simulink model "stm32f4_clcd_demo_4lines"  (Simulink 7.3)
settings: Solver=FixedStepDiscrete  SolverMode=SingleTasking  StartTime=0.0  StopTime=10.0  RelTol=1e-3
PreLoadFcn:
  | waijung.modelPreload; % Required for working with Waijung Blockset. Do not remove.
undefined symbols (not defined in the file): HSEOSC, Link, LQFP176, ST, STM32F417IG
libraries: simulink x1, stm32f4_adc_lib x1, stm32f4_device_config_lib x1
CloseFcn:
  | waijung.modelClose; % Required for working with Waijung Blockset. Do not remove.
settings Model: Creator=Krisada  LastModifiedBy=Krisada
settings OptimizationCC: OptimizeModelRefInitCode=on  LifeSpan=1
settings DebuggingCC: ParameterPrecisionLossMsg=none
settings HardwareCC: ProdEndianess=LittleEndian  ProdHWDeviceType=ARM Compatible->Cortex - M4  TargetEndianess=LittleEndian  TargetHWDeviceType=ARM Compatible->Cortex - M4
settings RTWCC: SystemTargetFile=stm32f4.tlc  GenerateMakefile=off  TemplateMakefile=ert_default_tmf  Description=STM32F4 Target  ProcessScript=stm32f4_make_rtw_hook
settings CodeAppCC: IgnoreCustomStorageClasses=off
settings STFCustomTargetCC: ModelReferenceCompliant=off  CombineOutputUpdateFcns=on  ERTCustomFileBanners=on  SupportContinuousTime=off  SupportNonInlinedSFcns=off  SystemTargetFile=stm32f4.tlc
settings ERTTargetCC: MultiwordLength=2048  ModelReferenceCompliant=off  ParMdlRefBuildCompliant=off  CompOptLevelCompliant=off  ERTFirstTimeCompliant=off  ModelStepFunctionPrototypeControlCompliant=off  CPPClassGenCompliant=off  ExtModeMexFile=noextcomm  InlinedParameterPlacement=NonHierarchical  ERTSrcFileBannerTemplate=stm32f4_code_template.cgt  ERTHdrFileBannerTemplate=stm32f4_code_template.cgt  ERTDataSrcFileTemplate=stm32f4_code_template.cgt  ERTDataHdrFileTemplate=stm32f4_code_template.cgt  ERTCustomFileTemplate=stm32f4_file_process.tlc

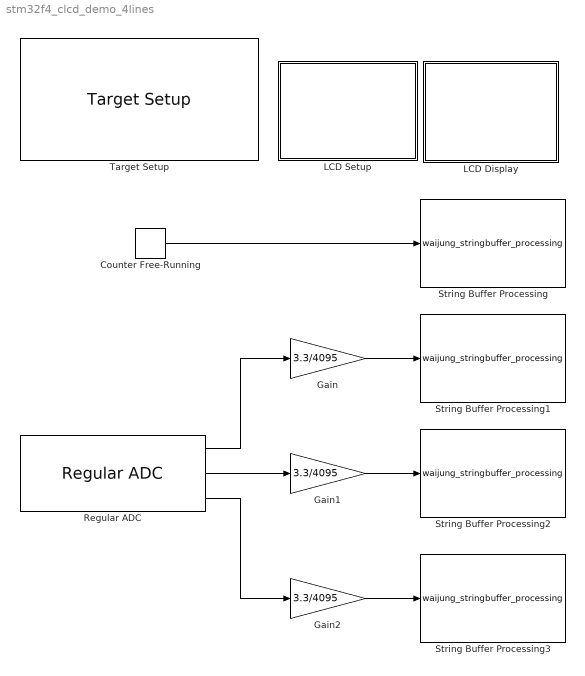
== system stm32f4_clcd_demo_4lines ==
  Counter Free-Running : simulink/Sources/Counter Free-Running  SystemSampleTime=-1  NumBits=16  tsamp=0.01
  Gain : Gain  Gain=3.3/4095  ParameterDataTypeMode=single  ParameterDataType=fixdt(1, 16)  ParameterScaling=2^0  ParamDataTypeStr=single  OutDataTypeMode=single  OutDataType=fixdt(1, 16)  OutScaling=2^0  OutDataTypeStr=single
  Gain1 : Gain  Gain=3.3/4095  ParameterDataTypeMode=single  ParameterDataType=fixdt(1, 16)  ParameterScaling=2^0  ParamDataTypeStr=single  OutDataTypeMode=single  OutDataType=fixdt(1, 16)  OutScaling=2^0  OutDataTypeStr=single
  Gain2 : Gain  Gain=3.3/4095  ParameterDataTypeMode=single  ParameterDataType=fixdt(1, 16)  ParameterScaling=2^0  ParamDataTypeStr=single  OutDataTypeMode=single  OutDataType=fixdt(1, 16)  OutScaling=2^0  OutDataTypeStr=single
  LCD Display : Subsystem
  LCD Setup : Subsystem
  Regular ADC : stm32f4_adc_lib/Regular ADC  adcmodule=1  outputdatatype=Single  prescaler=2  prescalerstr=ADC_Prescaler_Div2  chsamplingtime=Auto  chsamplingtimestr=ADC_SampleTime_480Cycles  read_an0=on  read_an1=on  read_an2=on  read_an3=off  read_an4=off  read_an5=off  read_an6=off  read_an7=off  read_an8=off  read_an9=off  read_an10=off  read_an11=off  read_an12=off  read_an13=off  read_an14=off  read_an15=off  read_an16=off  read_an17=off  read_an18=off  pinstr=GPIO_Pin_0 | GPIO_Pin_1 | GPIO_Pin_2  usedpinarray="[1  1  1  0  0  0  0  0  0  0  0  0  0  0  0  0  0  0  0]"  usedportidarray="[0  0  0]"  usedpinidarray="[0  1  2]"  usedpinidcount=3  sampletime=0.01  blockid=RegularADC  enablecustomportlabel=off  cinputportlabel=0  coutputportlabel=Out1, Out2
  String Buffer Processing : S-Function  FunctionName=waijung_stringbuffer_processing  Parameters=configuration,varname,sformat,porttypes,portcount,inputtypearray,outputtypearray,sampletime,sampletimestr,blockid  EnableBusSupport=off  mask(waijung_stringbuffer_processing){configuration=sprintf, storagename=Line1, sformat='Index: %u', enableoutput=off, varname=LCDSetupVolatileDataStorage_Line1, inputtypearray=[1 -1], outputtypearray=[0], porttypes=["uint32_t"], portcount=1, sampletime=-1, sampletimestr=0.01, blockid=StringBufferProcessing}
      mask prompts: configuration "Function"; storagename "String buffer"; sformat "Printf format"; enableoutput "Enable output status"; varname "Variable name"; inputtypearray "Input type array"; outputtypearray "Output type array"; porttypes "Port type list"; portcount "Port type count"; sampletime "Sample time (sec)"; sampletimestr "Compiled sample time (sec) in string"
      mask help:
      | This block implements string processing, sprintf/ sscanf command.
      | Supported format:
      | %u, %i, %o, %x: uint32
      | %d: int32
      | %e, %g, %f: single
      | %c: int8
      |
      | Status:
      |  0: Failed.
      |  Non-zero: Success.
      mask init:
      | waijung_stringbuffer_processing_callback('init');
      mask Help: web(fullfile(waijungdocroot,'String_Buffer_Processing.htm'))
      mask StyleString: popup(sprintf|sscanf),popup(Line1|Line2|Line3|Line4|<output>),edit,checkbox,edit,edit,edit,edit,edit,edit,edit,edit
      mask CallbackString: waijung_stringbuffer_processing_callback('configuration');||waijung_stringbuffer_processing_callback('sformat');|waijung_stringbuffer_processing_callback('enableoutput');||||||waijung_stringbuffer_processing_callback('sampletime');|waijung_stringbuffer_processing_callback('sampletimestr');|waijung_stringbuffer_processing_callback('blockid');
      mask Display: text(0.5, 0.5, '[ sprintf ]\nBuffer: Line1\nTs (sec): 0.01','ver','middle','hor','center');port_label('input', 1,'%u');
  String Buffer Processing1 : S-Function  FunctionName=waijung_stringbuffer_processing  Parameters=configuration,varname,sformat,porttypes,portcount,inputtypearray,outputtypearray,sampletime,sampletimestr,blockid  EnableBusSupport=off  mask(waijung_stringbuffer_processing){configuration=sprintf, storagename=Line2, sformat='AN0: %1.3f V', enableoutput=off, varname=LCDSetupVolatileDataStorage1_Line2, inputtypearray=[1 -1], outputtypearray=[0], porttypes=["float"], portcount=1, sampletime=-1, sampletimestr=0.01, blockid=StringBufferProcessing1}
      mask prompts: configuration "Function"; storagename "String buffer"; sformat "Printf format"; enableoutput "Enable output status"; varname "Variable name"; inputtypearray "Input type array"; outputtypearray "Output type array"; porttypes "Port type list"; portcount "Port type count"; sampletime "Sample time (sec)"; sampletimestr "Compiled sample time (sec) in string"
      mask help:
      | This block implements string processing, sprintf/ sscanf command.
      | Supported format:
      | %u, %i, %o, %x: uint32
      | %d: int32
      | %e, %g, %f: single
      | %c: int8
      |
      | Status:
      |  0: Failed.
      |  Non-zero: Success.
      mask init:
      | waijung_stringbuffer_processing_callback('init');
      mask Help: web(fullfile(waijungdocroot,'String_Buffer_Processing.htm'))
      mask StyleString: popup(sprintf|sscanf),popup(Line1|Line2|Line3|Line4|<output>),edit,checkbox,edit,edit,edit,edit,edit,edit,edit,edit
      mask CallbackString: waijung_stringbuffer_processing_callback('configuration');||waijung_stringbuffer_processing_callback('sformat');|waijung_stringbuffer_processing_callback('enableoutput');||||||waijung_stringbuffer_processing_callback('sampletime');|waijung_stringbuffer_processing_callback('sampletimestr');|waijung_stringbuffer_processing_callback('blockid');
      mask Display: text(0.5, 0.5, '[ sprintf ]\nBuffer: Line2\nTs (sec): 0.01','ver','middle','hor','center');port_label('input', 1,'%f');
  String Buffer Processing2 : S-Function  FunctionName=waijung_stringbuffer_processing  Parameters=configuration,varname,sformat,porttypes,portcount,inputtypearray,outputtypearray,sampletime,sampletimestr,blockid  EnableBusSupport=off  mask(waijung_stringbuffer_processing){configuration=sprintf, storagename=Line3, sformat='AN1: %1.3f V', enableoutput=off, varname=LCDSetupVolatileDataStorage2_Line3, inputtypearray=[1 -1], outputtypearray=[0], porttypes=["float"], portcount=1, sampletime=-1, sampletimestr=0.01, blockid=StringBufferProcessing2}
      mask prompts: configuration "Function"; storagename "String buffer"; sformat "Printf format"; enableoutput "Enable output status"; varname "Variable name"; inputtypearray "Input type array"; outputtypearray "Output type array"; porttypes "Port type list"; portcount "Port type count"; sampletime "Sample time (sec)"; sampletimestr "Compiled sample time (sec) in string"
      mask help:
      | This block implements string processing, sprintf/ sscanf command.
      | Supported format:
      | %u, %i, %o, %x: uint32
      | %d: int32
      | %e, %g, %f: single
      | %c: int8
      |
      | Status:
      |  0: Failed.
      |  Non-zero: Success.
      mask init:
      | waijung_stringbuffer_processing_callback('init');
      mask Help: web(fullfile(waijungdocroot,'String_Buffer_Processing.htm'))
      mask StyleString: popup(sprintf|sscanf),popup(Line1|Line2|Line3|Line4|<output>),edit,checkbox,edit,edit,edit,edit,edit,edit,edit,edit
      mask CallbackString: waijung_stringbuffer_processing_callback('configuration');||waijung_stringbuffer_processing_callback('sformat');|waijung_stringbuffer_processing_callback('enableoutput');||||||waijung_stringbuffer_processing_callback('sampletime');|waijung_stringbuffer_processing_callback('sampletimestr');|waijung_stringbuffer_processing_callback('blockid');
      mask Display: text(0.5, 0.5, '[ sprintf ]\nBuffer: Line3\nTs (sec): 0.01','ver','middle','hor','center');port_label('input', 1,'%f');
  String Buffer Processing3 : S-Function  FunctionName=waijung_stringbuffer_processing  Parameters=configuration,varname,sformat,porttypes,portcount,inputtypearray,outputtypearray,sampletime,sampletimestr,blockid  EnableBusSupport=off  mask(waijung_stringbuffer_processing){configuration=sprintf, storagename=Line4, sformat='AN2: %1.3f V', enableoutput=off, varname=LCDSetupVolatileDataStorage3_Line4, inputtypearray=[1 -1], outputtypearray=[0], porttypes=["float"], portcount=1, sampletime=-1, sampletimestr=0.01, blockid=StringBufferProcessing3}
      mask prompts: configuration "Function"; storagename "String buffer"; sformat "Printf format"; enableoutput "Enable output status"; varname "Variable name"; inputtypearray "Input type array"; outputtypearray "Output type array"; porttypes "Port type list"; portcount "Port type count"; sampletime "Sample time (sec)"; sampletimestr "Compiled sample time (sec) in string"
      mask help:
      | This block implements string processing, sprintf/ sscanf command.
      | Supported format:
      | %u, %i, %o, %x: uint32
      | %d: int32
      | %e, %g, %f: single
      | %c: int8
      |
      | Status:
      |  0: Failed.
      |  Non-zero: Success.
      mask init:
      | waijung_stringbuffer_processing_callback('init');
      mask Help: web(fullfile(waijungdocroot,'String_Buffer_Processing.htm'))
      mask StyleString: popup(sprintf|sscanf),popup(Line1|Line2|Line3|Line4|<output>),edit,checkbox,edit,edit,edit,edit,edit,edit,edit,edit
      mask CallbackString: waijung_stringbuffer_processing_callback('configuration');||waijung_stringbuffer_processing_callback('sformat');|waijung_stringbuffer_processing_callback('enableoutput');||||||waijung_stringbuffer_processing_callback('sampletime');|waijung_stringbuffer_processing_callback('sampletimestr');|waijung_stringbuffer_processing_callback('blockid');
      mask Display: text(0.5, 0.5, '[ sprintf ]\nBuffer: Line4\nTs (sec): 0.01','ver','middle','hor','center');port_label('input', 1,'%f');
  Target Setup : stm32f4_device_config_lib/Target Setup  Priority=100  compiler=GNU ARM  previous_compiler=GNU ARM  mcu=STM32F417IG (LQFP176)  mcustr=STM32F417IG  clockconfig=HSEOSC-8MHz  system_stm32f4xx_c_path=F:\trunk\targets\stm32f4_target\stm32f4\utils\system_stm32f4xx_default\STM32F40_41xxx\hseosc8mhz  showmemoryconfiguration=off  stacksize=0x400  heapsize=0x200  enableautocompiledownload=on  fullchiperase=off  programmerinterface=ST-Link  editctrlstr=on  compilercontrolstr=$(patsubst %, -I%, .) -mcpu=cortex-m4 -mthumb -mthumb-interwork -mfloat-abi=hard -mfpu=fpv4-sp-d16 -ffast-math -Wall -Wextra -Ofast  assemblercontrolstr=$(patsubst %, -I%, .) -mcpu=cortex-m4 -mthumb -mthumb-interwork -mfloat-abi=hard -mfpu=fpv4-sp-d16 -ffast-math -Wall -Wextra -Ofast -Wa,-amhls=$(<:.s=.lst) -D__STACK_SIZE=$(STACK_SIZE) -D__HEAP_SIZE=$(HEAP_SIZE)  linkercontrolstr=-T$(LD_SCRIPT) -g -Wl,-Map=$(MAP),--cref,--no-warn-mismatch -mcpu=cortex-m4 -mthumb -mthumb-interwork -mfloat-abi=hard -mfpu=fpv4-sp-d16 -specs=nosys.specs  runafterdownload=on  execprofile=None  profileruart=1  profilerbaud=115200  profilertxpin=D8  profilerinitstr=0.01,168000000,1680000,115200,0  manualsetsampletime=off  sampletime=0.01  blockid=TargetSetup  systickreloadvalue=1680000  hseval=8000000  lastprofileruart=1  hclk=168000000  flashorigin=0x8000000  flashlength=1024k  ramorigin=0x20000000  ramlength=128k  useextram=off
  wires:
  Gain/1 -> String Buffer Processing1/1
  Counter Free-Running/1 -> String Buffer Processing/1
  Gain1/1 -> String Buffer Processing2/1
  Gain2/1 -> String Buffer Processing3/1
  Regular ADC/1 -> Gain/1
  Regular ADC/2 -> Gain1/1
  Regular ADC/3 -> Gain2/1

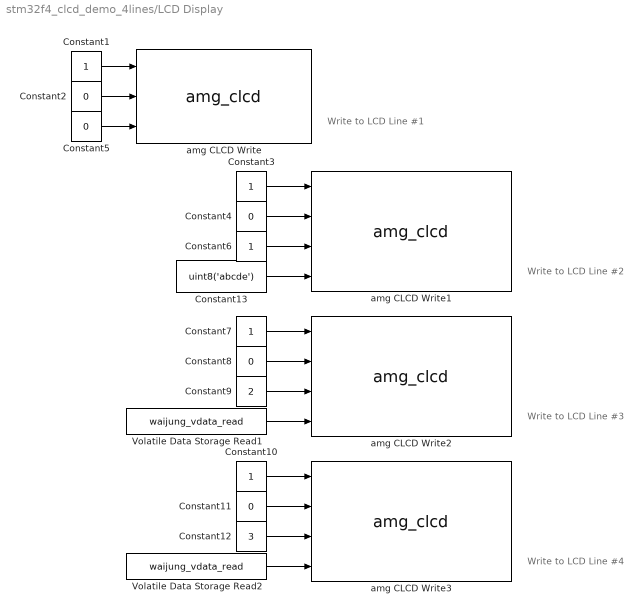
== system stm32f4_clcd_demo_4lines/LCD Display ==
  note: Write to LCD Line #1
  note: Write to LCD Line #2
  note: Write to LCD Line #3
  note: Write to LCD Line #4
  Constant{1,3,6..7,10} (5 alike) : Constant  OutDataTypeMode=uint8  OutDataType=fixdt(1, 16)  OutScaling=2^0  OutDataTypeStr=uint8
  Constant{2,4..5,8,11} (5 alike) : Constant  Value=0  OutDataTypeMode=uint8  OutDataType=fixdt(1, 16)  OutScaling=2^0  OutDataTypeStr=uint8
  Constant12 : Constant  Value=3  OutDataTypeMode=uint8  OutDataType=fixdt(1, 16)  OutScaling=2^0  OutDataTypeStr=uint8
  Constant13 : Constant  Value=uint8('abcde')  OutDataTypeMode=uint8  OutDataType=fixdt(1, 16)  OutScaling=2^0  OutDataTypeStr=uint8
  Constant9 : Constant  Value=2  OutDataTypeMode=uint8  OutDataType=fixdt(1, 16)  OutScaling=2^0  OutDataTypeStr=uint8
  Volatile Data Storage Read1 : S-Function  FunctionName=waijung_vdata_read  Parameters=storagename,varname,sampletime,sampletimestr,blockid,storagetype,storagetypestr  EnableBusSupport=off  mask(waijung_vdata_read){storagename=Line3, varname=LCDSetupVolatileDataStorage2_Line3, sampletime=inf, sampletimestr=0.01, blockid=LCDDisplayVolatileDataStorageRead1, storagetype=string, storagetypestr=uint32_t}
      mask prompts: storagename "Storage Name"; varname "Variable name"; sampletime "Sample time (sec)"; sampletimestr "Compiled sample time (sec) in string"; storagetype "Data type"; storagetypestr "Data type string"
      mask help: This block implements read data from a buffer.
      mask init:
      | waijung_vdata_read_callback('init');
      mask Help: web(fullfile(waijungdocroot,'waijung_vdata_read.htm'))
      mask StyleString: popup(Line1|Line2|Line3|Line4),edit,edit,edit,edit,edit,edit
      mask CallbackString: waijung_vdata_read_callback('storagename');|waijung_vdata_read_callback('varname');|waijung_vdata_read_callback('sampletime');|waijung_vdata_read_callback('sampletimestr');|waijung_vdata_read_callback('blockid');|waijung_vdata_read_callback('storagetype');|
      mask Display: text(0.05, 0.5, 'Buffer: Line3','ver','middle','hor','left');port_label('output',1,'D1(string)')
  Volatile Data Storage Read2 : S-Function  FunctionName=waijung_vdata_read  Parameters=storagename,varname,sampletime,sampletimestr,blockid,storagetype,storagetypestr  EnableBusSupport=off  mask(waijung_vdata_read){storagename=Line4, varname=LCDSetupVolatileDataStorage3_Line4, sampletime=inf, sampletimestr=0.01, blockid=LCDDisplayVolatileDataStorageRead2, storagetype=string, storagetypestr=uint32_t}
      mask prompts: storagename "Storage Name"; varname "Variable name"; sampletime "Sample time (sec)"; sampletimestr "Compiled sample time (sec) in string"; storagetype "Data type"; storagetypestr "Data type string"
      mask help: This block implements read data from a buffer.
      mask init:
      | waijung_vdata_read_callback('init');
      mask Help: web(fullfile(waijungdocroot,'waijung_vdata_read.htm'))
      mask StyleString: popup(Line1|Line2|Line3|Line4),edit,edit,edit,edit,edit,edit
      mask CallbackString: waijung_vdata_read_callback('storagename');|waijung_vdata_read_callback('varname');|waijung_vdata_read_callback('sampletime');|waijung_vdata_read_callback('sampletimestr');|waijung_vdata_read_callback('blockid');|waijung_vdata_read_callback('storagetype');|
      mask Display: text(0.05, 0.5, 'Buffer: Line4','ver','middle','hor','left');port_label('output',1,'D1(string)')
  amg CLCD Write : S-Function  FunctionName=amg_clcd  Parameters=module,configuration,inputtypearray,outputtypearray,confstr,sampletime,sampletimestr,blockid  EnableBusSupport=off  mask(amg_clcd){configuration=Transaction, module=1, model=amg CLCD Std, interface=4-bits, linecount=4, columncount=20, gpiotype=Push-pull, controlport=E, control_rs=15, control_en=11, control_rw=13, dataport=A, data0=7, data1=5, data2=3, data3=1, usestringbuffer=on, stringbuffer=Line1, varname=LCDSetupVolatileDataStorage_Line1, inputtypearray=[3 -1 -1 -1], outputtypearray=[0], confstr=["4","4","20","PP","E","15","11","13","","A","","","","","7","5","3","1","1","LCDSetupVolatileDataStorage_Line1","1","0","0","0","1","0","0","0","0","stm32f4"], sampletime=0.01, sampletimestr=0.01, blockid=LCDDisplayamgCLCDWrite}
      mask prompts: model "LCD model:"; linecount "Number of lines:"; columncount "Number of columns:"; gpiotype "GPIO Pull-Up/Down:"; controlport "GPIO control port:"; control_rs "GPIO control pin, RS:"; control_en "GPIO control pin, EN:"; control_rw "GPIO control pin, RW:"; dataport "GPIO data D[7:4] port"; data0 "GPIO data pin, D4:"; data1 "GPIO data pin, D5:"; data2 "GPIO data pin, D6:"; data3 "GPIO data pin, D7:"; usestringbuffer "Use string buffer"; stringbuffer "String buffer"; varname "Variable name"; inputtypearray "Input type array"; outputtypearray "Output type array"; confstr "Configuration string"; sampletime "Sample time (sec)"; sampletimestr "Compiled sample time (sec) in string"
      mask help:
      | Note for cmd:
      | 1 - Clear LCD Line before write.
      | 0 or otherwise - Write into LCD Line with existing data.
      mask init:
      | amg_clcd_callback('init');
      mask Help: web(fullfile(waijungdocroot,'amg_clcd_write.htm'), '-browser')
      mask StyleString: popup(Setup|Transaction),popup(1|2|3|4),popup(amg CLCD Std),popup(4-bits),edit,edit,popup(Push-pull|Open-drain),popup(A|B|C|D|E|F|G|H|I),popup(0|1|2|3|4|5|6|7|8|9|10|11|12|13|14|15),popup(0|1|2|3|4|5|6|7|8|9|10|11|12|13|14|15),popup(0|1|2|3|4|5|6|7|8|9|10|11|12|13|14|15),popup(A|B|C|D|E|F|G|H|I),popup(0|1|2|3|4|5|6|7|8|9|10|11|12|13|14|15),popup(0|1|2|3|4|5|6|7|8|9|10|11|12|13|14|15),popup(0|1|2|3|4|5|6|7|8|9|10|11|12|13|14|15),popup(0|1|2|3|4|5|6|7|8|9|10|11|12|13|14|15),checkbox,popup(Line1|Line2|Line3|Line4),edit,edit,edit,edit,edit,edit,edit
      mask CallbackString: amg_clcd_callback('configuration');||||||||||||||||amg_clcd_callback('usestringbuffer');||amg_clcd_callback('varname');|||amg_clcd_callback('confstr');|amg_clcd_callback('sampletime');|amg_clcd_callback('sampletimestr');|amg_clcd_callback('blockid');
      mask Display: text(0.5, 0.5, 'Module: CLCD1 (Write)\nBuffer: Line1\nTs (sec): 0.01','ver','middle','hor','center');port_label('input', 1,'cmd');port_label('input', 2,'xpos');port_label('input', 3,'ypos');
  amg CLCD Write1 : S-Function  FunctionName=amg_clcd  Parameters=module,configuration,inputtypearray,outputtypearray,confstr,sampletime,sampletimestr,blockid  EnableBusSupport=off  mask(amg_clcd){configuration=Transaction, module=1, model=amg CLCD Std, interface=4-bits, linecount=4, columncount=20, gpiotype=Push-pull, controlport=E, control_rs=15, control_en=11, control_rw=13, dataport=A, data0=7, data1=5, data2=3, data3=1, usestringbuffer=off, stringbuffer=Line2, varname=LCDSetupVolatileDataStorage1_Line2, inputtypearray=[4 -1 -1 -1 -1], outputtypearray=[0], confstr=["4","4","20","PP","E","15","11","13","","A","","","","","7","5","3","1","0","","1","0","0","0","1","0","0","0","0","stm32f4"], sampletime=0.01, sampletimestr=0.01, blockid=LCDDisplayamgCLCDWrite1}
      mask prompts: model "LCD model:"; linecount "Number of lines:"; columncount "Number of columns:"; gpiotype "GPIO Pull-Up/Down:"; controlport "GPIO control port:"; control_rs "GPIO control pin, RS:"; control_en "GPIO control pin, EN:"; control_rw "GPIO control pin, RW:"; dataport "GPIO data D[7:4] port"; data0 "GPIO data pin, D4:"; data1 "GPIO data pin, D5:"; data2 "GPIO data pin, D6:"; data3 "GPIO data pin, D7:"; usestringbuffer "Use string buffer"; stringbuffer "String buffer"; varname "Variable name"; inputtypearray "Input type array"; outputtypearray "Output type array"; confstr "Configuration string"; sampletime "Sample time (sec)"; sampletimestr "Compiled sample time (sec) in string"
      mask help:
      | Note for cmd:
      | 1 - Clear LCD Line before write.
      | 0 or otherwise - Write into LCD Line with existing data.
      mask init:
      | amg_clcd_callback('init');
      mask Help: web(fullfile(waijungdocroot,'amg_clcd_write.htm'), '-browser')
      mask StyleString: popup(Setup|Transaction),popup(1|2|3|4),popup(amg CLCD Std),popup(4-bits),edit,edit,popup(Push-pull|Open-drain),popup(A|B|C|D|E|F|G|H|I),popup(0|1|2|3|4|5|6|7|8|9|10|11|12|13|14|15),popup(0|1|2|3|4|5|6|7|8|9|10|11|12|13|14|15),popup(0|1|2|3|4|5|6|7|8|9|10|11|12|13|14|15),popup(A|B|C|D|E|F|G|H|I),popup(0|1|2|3|4|5|6|7|8|9|10|11|12|13|14|15),popup(0|1|2|3|4|5|6|7|8|9|10|11|12|13|14|15),popup(0|1|2|3|4|5|6|7|8|9|10|11|12|13|14|15),popup(0|1|2|3|4|5|6|7|8|9|10|11|12|13|14|15),checkbox,popup(Line1|Line2|Line3|Line4),edit,edit,edit,edit,edit,edit,edit
      mask CallbackString: amg_clcd_callback('configuration');||||||||||||||||amg_clcd_callback('usestringbuffer');||amg_clcd_callback('varname');|||amg_clcd_callback('confstr');|amg_clcd_callback('sampletime');|amg_clcd_callback('sampletimestr');|amg_clcd_callback('blockid');
      mask Display: text(0.5, 0.5, 'Module: CLCD1 (Write)\nTs (sec): 0.01','ver','middle','hor','center');port_label('input', 1,'cmd');port_label('input', 2,'xpos');port_label('input', 3,'ypos');port_label('input', 4,'str');
  amg CLCD Write2 : S-Function  FunctionName=amg_clcd  Parameters=module,configuration,inputtypearray,outputtypearray,confstr,sampletime,sampletimestr,blockid  EnableBusSupport=off  mask(amg_clcd){configuration=Transaction, module=1, model=amg CLCD Std, interface=4-bits, linecount=4, columncount=20, gpiotype=Push-pull, controlport=E, control_rs=15, control_en=11, control_rw=13, dataport=A, data0=7, data1=5, data2=3, data3=1, usestringbuffer=off, stringbuffer=Line2, varname=LCDSetupVolatileDataStorage1_Line2, inputtypearray=[4 -1 -1 -1 -1], outputtypearray=[0], confstr=["4","4","20","PP","E","15","11","13","","A","","","","","7","5","3","1","0","","1","0","0","0","1","0","0","0","0","stm32f4"], sampletime=0.01, sampletimestr=0.01, blockid=LCDDisplayamgCLCDWrite2}
      mask prompts: model "LCD model:"; linecount "Number of lines:"; columncount "Number of columns:"; gpiotype "GPIO Pull-Up/Down:"; controlport "GPIO control port:"; control_rs "GPIO control pin, RS:"; control_en "GPIO control pin, EN:"; control_rw "GPIO control pin, RW:"; dataport "GPIO data D[7:4] port"; data0 "GPIO data pin, D4:"; data1 "GPIO data pin, D5:"; data2 "GPIO data pin, D6:"; data3 "GPIO data pin, D7:"; usestringbuffer "Use string buffer"; stringbuffer "String buffer"; varname "Variable name"; inputtypearray "Input type array"; outputtypearray "Output type array"; confstr "Configuration string"; sampletime "Sample time (sec)"; sampletimestr "Compiled sample time (sec) in string"
      mask help:
      | Note for cmd:
      | 1 - Clear LCD Line before write.
      | 0 or otherwise - Write into LCD Line with existing data.
      mask init:
      | amg_clcd_callback('init');
      mask Help: web(fullfile(waijungdocroot,'amg_clcd_write.htm'), '-browser')
      mask StyleString: popup(Setup|Transaction),popup(1|2|3|4),popup(amg CLCD Std),popup(4-bits),edit,edit,popup(Push-pull|Open-drain),popup(A|B|C|D|E|F|G|H|I),popup(0|1|2|3|4|5|6|7|8|9|10|11|12|13|14|15),popup(0|1|2|3|4|5|6|7|8|9|10|11|12|13|14|15),popup(0|1|2|3|4|5|6|7|8|9|10|11|12|13|14|15),popup(A|B|C|D|E|F|G|H|I),popup(0|1|2|3|4|5|6|7|8|9|10|11|12|13|14|15),popup(0|1|2|3|4|5|6|7|8|9|10|11|12|13|14|15),popup(0|1|2|3|4|5|6|7|8|9|10|11|12|13|14|15),popup(0|1|2|3|4|5|6|7|8|9|10|11|12|13|14|15),checkbox,popup(Line1|Line2|Line3|Line4),edit,edit,edit,edit,edit,edit,edit
      mask CallbackString: amg_clcd_callback('configuration');||||||||||||||||amg_clcd_callback('usestringbuffer');||amg_clcd_callback('varname');|||amg_clcd_callback('confstr');|amg_clcd_callback('sampletime');|amg_clcd_callback('sampletimestr');|amg_clcd_callback('blockid');
      mask Display: text(0.5, 0.5, 'Module: CLCD1 (Write)\nTs (sec): 0.01','ver','middle','hor','center');port_label('input', 1,'cmd');port_label('input', 2,'xpos');port_label('input', 3,'ypos');port_label('input', 4,'str');
  amg CLCD Write3 : S-Function  FunctionName=amg_clcd  Parameters=module,configuration,inputtypearray,outputtypearray,confstr,sampletime,sampletimestr,blockid  EnableBusSupport=off  mask(amg_clcd){configuration=Transaction, module=1, model=amg CLCD Std, interface=4-bits, linecount=4, columncount=20, gpiotype=Push-pull, controlport=E, control_rs=15, control_en=11, control_rw=13, dataport=A, data0=7, data1=5, data2=3, data3=1, usestringbuffer=off, stringbuffer=Line2, varname=LCDSetupVolatileDataStorage1_Line2, inputtypearray=[4 -1 -1 -1 -1], outputtypearray=[0], confstr=["4","4","20","PP","E","15","11","13","","A","","","","","7","5","3","1","0","","1","0","0","0","1","0","0","0","0","stm32f4"], sampletime=0.01, sampletimestr=0.01, blockid=LCDDisplayamgCLCDWrite3}
      mask prompts: model "LCD model:"; linecount "Number of lines:"; columncount "Number of columns:"; gpiotype "GPIO Pull-Up/Down:"; controlport "GPIO control port:"; control_rs "GPIO control pin, RS:"; control_en "GPIO control pin, EN:"; control_rw "GPIO control pin, RW:"; dataport "GPIO data D[7:4] port"; data0 "GPIO data pin, D4:"; data1 "GPIO data pin, D5:"; data2 "GPIO data pin, D6:"; data3 "GPIO data pin, D7:"; usestringbuffer "Use string buffer"; stringbuffer "String buffer"; varname "Variable name"; inputtypearray "Input type array"; outputtypearray "Output type array"; confstr "Configuration string"; sampletime "Sample time (sec)"; sampletimestr "Compiled sample time (sec) in string"
      mask help:
      | Note for cmd:
      | 1 - Clear LCD Line before write.
      | 0 or otherwise - Write into LCD Line with existing data.
      mask init:
      | amg_clcd_callback('init');
      mask Help: web(fullfile(waijungdocroot,'amg_clcd_write.htm'), '-browser')
      mask StyleString: popup(Setup|Transaction),popup(1|2|3|4),popup(amg CLCD Std),popup(4-bits),edit,edit,popup(Push-pull|Open-drain),popup(A|B|C|D|E|F|G|H|I),popup(0|1|2|3|4|5|6|7|8|9|10|11|12|13|14|15),popup(0|1|2|3|4|5|6|7|8|9|10|11|12|13|14|15),popup(0|1|2|3|4|5|6|7|8|9|10|11|12|13|14|15),popup(A|B|C|D|E|F|G|H|I),popup(0|1|2|3|4|5|6|7|8|9|10|11|12|13|14|15),popup(0|1|2|3|4|5|6|7|8|9|10|11|12|13|14|15),popup(0|1|2|3|4|5|6|7|8|9|10|11|12|13|14|15),popup(0|1|2|3|4|5|6|7|8|9|10|11|12|13|14|15),checkbox,popup(Line1|Line2|Line3|Line4),edit,edit,edit,edit,edit,edit,edit
      mask CallbackString: amg_clcd_callback('configuration');||||||||||||||||amg_clcd_callback('usestringbuffer');||amg_clcd_callback('varname');|||amg_clcd_callback('confstr');|amg_clcd_callback('sampletime');|amg_clcd_callback('sampletimestr');|amg_clcd_callback('blockid');
      mask Display: text(0.5, 0.5, 'Module: CLCD1 (Write)\nTs (sec): 0.01','ver','middle','hor','center');port_label('input', 1,'cmd');port_label('input', 2,'xpos');port_label('input', 3,'ypos');port_label('input', 4,'str');
  wires:
  Constant1/1 -> amg CLCD Write/1
  Constant3/1 -> amg CLCD Write1/1
  Constant4/1 -> amg CLCD Write1/2
  Constant13/1 -> amg CLCD Write1/4
  Constant2/1 -> amg CLCD Write/2
  Constant5/1 -> amg CLCD Write/3
  Constant6/1 -> amg CLCD Write1/3
  Constant7/1 -> amg CLCD Write2/1
  Constant8/1 -> amg CLCD Write2/2
  Volatile Data Storage Read1/1 -> amg CLCD Write2/4
  Constant9/1 -> amg CLCD Write2/3
  Constant10/1 -> amg CLCD Write3/1
  Constant11/1 -> amg CLCD Write3/2
  Volatile Data Storage Read2/1 -> amg CLCD Write3/4
  Constant12/1 -> amg CLCD Write3/3

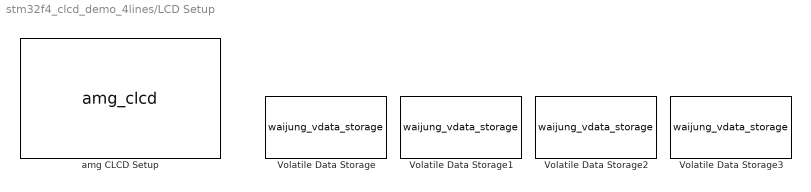
== system stm32f4_clcd_demo_4lines/LCD Setup ==
  Volatile Data Storage : S-Function  FunctionName=waijung_vdata_storage  Parameters=storagetype,storagename,initval,varname,buffersize,initvalstring,sampletime,sampletimestr,blockid,storagetypestr  EnableBusSupport=off  mask(waijung_vdata_storage){storagetype=string, storagename=Line1, initval=0, varname=LCDSetupVolatileDataStorage_Line1, buffersize=64, initvalstring='', webintegration=Disable, weboutputformat='%s', webcgicallback=(void*)0, laststoragetype=string, sampletime=-1, sampletimestr=0.01, blockid=LCDSetupVolatileDataStorage, storagetypestr=char}
      mask prompts: storagetype "Storage Type"; storagename "Storage Name (must be a valid variable name)"; initval "Initial value (Apply at Power on Reset only)"; varname "Variable name"; buffersize "Size (bytes)"; initvalstring "Initial value (Apply at Power on Reset only)"; webintegration "Web CGI varget/varset integration"; weboutputformat "Web CGI varget output format"; webcgicallback "Web CGI varset callback"; laststoragetype "Last selected Storage Type"; sampletime "Sample time (sec)"; sampletimestr "Compiled sample time (sec) in string"; storagetypestr "Type string"
      mask help:
      | This block implements a volatile Data Storage.
      |
      | Web CGI varset/varget integratiopn:
      | Enable - In webserver application, allow remote access via http.
      | Disable - Variable is use in local only.
      mask init:
      | waijung_vdata_storage_callback('init');
      mask Help: web(fullfile(waijungdocroot,'Volatile_Data_Storage.htm'))
      mask StyleString: popup(double|single|uint32|int32|uint16|int16|uint8|int8|string),edit,edit,edit,edit,edit,popup(Disable|ReadOnly|Write/ Read|ReadOnly with KeyValuePair|Write/ Read with KeyValuePair),edit,edit,popup(double|single|uint32|int32|uint16|int16|uint8|int8|string),edit,edit,edit,edit
      mask CallbackString: waijung_vdata_storage_callback('storagetype');|waijung_vdata_storage_callback('storagename');|waijung_vdata_storage_callback('initval');|waijung_vdata_storage_callback('varname');||waijung_vdata_storage_callback('initvalstring');|waijung_vdata_storage_callback('webintegration');|waijung_vdata_storage_callback('weboutputformat');|||waijung_vdata_storage_callback('sampletime');|waijung_vdata_storage_callback('sampletimestr');|waijung_vdata_storage_callback('blockid');|
      mask Display: text(0.5, 0.5, 'Name: Line1\nType: string','ver','middle','hor','center')
  Volatile Data Storage1 : S-Function  FunctionName=waijung_vdata_storage  Parameters=storagetype,storagename,initval,varname,buffersize,initvalstring,sampletime,sampletimestr,blockid,storagetypestr  EnableBusSupport=off  mask(waijung_vdata_storage){storagetype=string, storagename=Line2, initval=0, varname=LCDSetupVolatileDataStorage1_Line2, buffersize=64, initvalstring='', webintegration=Disable, weboutputformat='%s', webcgicallback=(void*)0, laststoragetype=string, sampletime=-1, sampletimestr=0.01, blockid=LCDSetupVolatileDataStorage1, storagetypestr=char}
      mask prompts: storagetype "Storage Type"; storagename "Storage Name (must be a valid variable name)"; initval "Initial value (Apply at Power on Reset only)"; varname "Variable name"; buffersize "Size (bytes)"; initvalstring "Initial value (Apply at Power on Reset only)"; webintegration "Web CGI varget/varset integration"; weboutputformat "Web CGI varget output format"; webcgicallback "Web CGI varset callback"; laststoragetype "Last selected Storage Type"; sampletime "Sample time (sec)"; sampletimestr "Compiled sample time (sec) in string"; storagetypestr "Type string"
      mask help:
      | This block implements a volatile Data Storage.
      |
      | Web CGI varset/varget integratiopn:
      | Enable - In webserver application, allow remote access via http.
      | Disable - Variable is use in local only.
      mask init:
      | waijung_vdata_storage_callback('init');
      mask Help: web(fullfile(waijungdocroot,'Volatile_Data_Storage.htm'))
      mask StyleString: popup(double|single|uint32|int32|uint16|int16|uint8|int8|string),edit,edit,edit,edit,edit,popup(Disable|ReadOnly|Write/ Read|ReadOnly with KeyValuePair|Write/ Read with KeyValuePair),edit,edit,popup(double|single|uint32|int32|uint16|int16|uint8|int8|string),edit,edit,edit,edit
      mask CallbackString: waijung_vdata_storage_callback('storagetype');|waijung_vdata_storage_callback('storagename');|waijung_vdata_storage_callback('initval');|waijung_vdata_storage_callback('varname');||waijung_vdata_storage_callback('initvalstring');|waijung_vdata_storage_callback('webintegration');|waijung_vdata_storage_callback('weboutputformat');|||waijung_vdata_storage_callback('sampletime');|waijung_vdata_storage_callback('sampletimestr');|waijung_vdata_storage_callback('blockid');|
      mask Display: text(0.5, 0.5, 'Name: Line2\nType: string','ver','middle','hor','center')
  Volatile Data Storage2 : S-Function  FunctionName=waijung_vdata_storage  Parameters=storagetype,storagename,initval,varname,buffersize,initvalstring,sampletime,sampletimestr,blockid,storagetypestr  EnableBusSupport=off  mask(waijung_vdata_storage){storagetype=string, storagename=Line3, initval=0, varname=LCDSetupVolatileDataStorage2_Line3, buffersize=64, initvalstring='', webintegration=Disable, weboutputformat='%s', webcgicallback=(void*)0, laststoragetype=string, sampletime=-1, sampletimestr=0.01, blockid=LCDSetupVolatileDataStorage2, storagetypestr=char}
      mask prompts: storagetype "Storage Type"; storagename "Storage Name (must be a valid variable name)"; initval "Initial value (Apply at Power on Reset only)"; varname "Variable name"; buffersize "Size (bytes)"; initvalstring "Initial value (Apply at Power on Reset only)"; webintegration "Web CGI varget/varset integration"; weboutputformat "Web CGI varget output format"; webcgicallback "Web CGI varset callback"; laststoragetype "Last selected Storage Type"; sampletime "Sample time (sec)"; sampletimestr "Compiled sample time (sec) in string"; storagetypestr "Type string"
      mask help:
      | This block implements a volatile Data Storage.
      |
      | Web CGI varset/varget integratiopn:
      | Enable - In webserver application, allow remote access via http.
      | Disable - Variable is use in local only.
      mask init:
      | waijung_vdata_storage_callback('init');
      mask Help: web(fullfile(waijungdocroot,'Volatile_Data_Storage.htm'))
      mask StyleString: popup(double|single|uint32|int32|uint16|int16|uint8|int8|string),edit,edit,edit,edit,edit,popup(Disable|ReadOnly|Write/ Read|ReadOnly with KeyValuePair|Write/ Read with KeyValuePair),edit,edit,popup(double|single|uint32|int32|uint16|int16|uint8|int8|string),edit,edit,edit,edit
      mask CallbackString: waijung_vdata_storage_callback('storagetype');|waijung_vdata_storage_callback('storagename');|waijung_vdata_storage_callback('initval');|waijung_vdata_storage_callback('varname');||waijung_vdata_storage_callback('initvalstring');|waijung_vdata_storage_callback('webintegration');|waijung_vdata_storage_callback('weboutputformat');|||waijung_vdata_storage_callback('sampletime');|waijung_vdata_storage_callback('sampletimestr');|waijung_vdata_storage_callback('blockid');|
      mask Display: text(0.5, 0.5, 'Name: Line3\nType: string','ver','middle','hor','center')
  Volatile Data Storage3 : S-Function  FunctionName=waijung_vdata_storage  Parameters=storagetype,storagename,initval,varname,buffersize,initvalstring,sampletime,sampletimestr,blockid,storagetypestr  EnableBusSupport=off  mask(waijung_vdata_storage){storagetype=string, storagename=Line4, initval=0, varname=LCDSetupVolatileDataStorage3_Line4, buffersize=64, initvalstring='', webintegration=Disable, weboutputformat='%s', webcgicallback=(void*)0, laststoragetype=string, sampletime=-1, sampletimestr=0.01, blockid=LCDSetupVolatileDataStorage3, storagetypestr=char}
      mask prompts: storagetype "Storage Type"; storagename "Storage Name (must be a valid variable name)"; initval "Initial value (Apply at Power on Reset only)"; varname "Variable name"; buffersize "Size (bytes)"; initvalstring "Initial value (Apply at Power on Reset only)"; webintegration "Web CGI varget/varset integration"; weboutputformat "Web CGI varget output format"; webcgicallback "Web CGI varset callback"; laststoragetype "Last selected Storage Type"; sampletime "Sample time (sec)"; sampletimestr "Compiled sample time (sec) in string"; storagetypestr "Type string"
      mask help:
      | This block implements a volatile Data Storage.
      |
      | Web CGI varset/varget integratiopn:
      | Enable - In webserver application, allow remote access via http.
      | Disable - Variable is use in local only.
      mask init:
      | waijung_vdata_storage_callback('init');
      mask Help: web(fullfile(waijungdocroot,'Volatile_Data_Storage.htm'))
      mask StyleString: popup(double|single|uint32|int32|uint16|int16|uint8|int8|string),edit,edit,edit,edit,edit,popup(Disable|ReadOnly|Write/ Read|ReadOnly with KeyValuePair|Write/ Read with KeyValuePair),edit,edit,popup(double|single|uint32|int32|uint16|int16|uint8|int8|string),edit,edit,edit,edit
      mask CallbackString: waijung_vdata_storage_callback('storagetype');|waijung_vdata_storage_callback('storagename');|waijung_vdata_storage_callback('initval');|waijung_vdata_storage_callback('varname');||waijung_vdata_storage_callback('initvalstring');|waijung_vdata_storage_callback('webintegration');|waijung_vdata_storage_callback('weboutputformat');|||waijung_vdata_storage_callback('sampletime');|waijung_vdata_storage_callback('sampletimestr');|waijung_vdata_storage_callback('blockid');|
      mask Display: text(0.5, 0.5, 'Name: Line4\nType: string','ver','middle','hor','center')
  amg CLCD Setup : S-Function  FunctionName=amg_clcd  Parameters=module,configuration,inputtypearray,outputtypearray,confstr,sampletime,sampletimestr,blockid  EnableBusSupport=off  mask(amg_clcd){configuration=Setup, module=1, model=amg CLCD Std, interface=4-bits, linecount=4, columncount=16, gpiotype=Push-pull, controlport=E, control_rs=7, control_rw=8, control_en=9, dataport=E, data0=12, data1=13, data2=14, data3=15, usestringbuffer=off, stringbuffer=Line2, varname=clcd_demo_4linesLCDSetupVolatileDataStorage3_Line2, inputtypearray=[0], outputtypearray=[0], confstr=["4","4","16","PP","E","7","9","8","","E","","","","","12","13","14","15","0","","0","0","0","0","1","0","0","0","0","stm32f4"], sampletime=-1, sampletimestr=0.01, blockid=LCDSetupamgCLCDSetup}
      mask prompts: model "LCD model:"; linecount "Number of lines:"; columncount "Number of columns:"; gpiotype "GPIO Pull-Up/Down:"; controlport "GPIO control port:"; control_rs "GPIO control pin, RS:"; control_rw "GPIO control pin, RW:"; control_en "GPIO control pin, EN:"; dataport "GPIO data D[7:4] port"; data0 "GPIO data pin, D4:"; data1 "GPIO data pin, D5:"; data2 "GPIO data pin, D6:"; data3 "GPIO data pin, D7:"; usestringbuffer "Use string buffer"; stringbuffer "String buffer"; varname "Variable name"; inputtypearray "Input type array"; outputtypearray "Output type array"; confstr "Configuration string"; sampletime "Sample time (sec)"; sampletimestr "Compiled sample time (sec) in string"
      mask init:
      | amg_clcd_callback('init');
      mask Help: web(fullfile(waijungdocroot,'amg_clcd_setup.htm'), '-browser')
      mask StyleString: popup(Setup|Transaction),popup(1|2|3|4),popup(amg CLCD Std),popup(4-bits),edit,edit,popup(Push-pull|Open-drain),popup(A|B|C|D|E|F|G|H|I),popup(0|1|2|3|4|5|6|7|8|9|10|11|12|13|14|15),popup(0|1|2|3|4|5|6|7|8|9|10|11|12|13|14|15),popup(0|1|2|3|4|5|6|7|8|9|10|11|12|13|14|15),popup(A|B|C|D|E|F|G|H|I),popup(0|1|2|3|4|5|6|7|8|9|10|11|12|13|14|15),popup(0|1|2|3|4|5|6|7|8|9|10|11|12|13|14|15),popup(0|1|2|3|4|5|6|7|8|9|10|11|12|13|14|15),popup(0|1|2|3|4|5|6|7|8|9|10|11|12|13|14|15),checkbox,popup(Line3|Line1|Line2|Line4),edit,edit,edit,edit,edit,edit,edit
      mask CallbackString: amg_clcd_callback('configuration');||||||||||||||||amg_clcd_callback('usestringbuffer');||amg_clcd_callback('varname');|||amg_clcd_callback('confstr');|amg_clcd_callback('sampletime');|amg_clcd_callback('sampletimestr');|amg_clcd_callback('blockid');
      mask Display: text(0.5, 0.5, 'Module: CLCD1 (Setup)\nInterface: 4-bits\nCntrl: E7/E8/E9\nD[7:4]: E12/E13/E14/E15\nTs (sec): 0.01','ver','middle','hor','center');
